simulink model "average_example"  (R2018b)
settings: Solver=ode45  StartTime=0.0  StopTime=24*3600  MaxStep=60  RelTol=1e-3  EnableMultiTasking=on
libraries: carnot x1
settings Model: Creator=drhf  LastModifiedBy=drhf
settings DataIOCC: LimitDataPoints=on  SaveFormat=Array  SignalLoggingSaveFormat=ModelDataLogs
settings OptimizationCC: ExpressionDepthLimit=2147483647  LifeSpan=inf
settings DebuggingCC: UnderspecifiedInitializationDetection=Classic  MergeDetectMultiDrivingBlocksExec=none  SolverPrmCheckMsg=warning  FcnCallInpInsideContextMsg=warning  StateNameClashWarn=warning  SFUnexpectedBacktrackingDiag=warning  SFNoUnconditionalDefaultTransitionDiag=warning  SFExecutionAtInitializationDiag=none
settings HardwareCC: ProdBitPerPointer=32  ProdBitPerSizeT=32  ProdBitPerPtrDiffT=32  ProdLargestAtomicFloat=None  ProdIntDivRoundTo=Undefined  ProdEndianess=Unspecified  ProdWordSize=32  ProdHWDeviceType=32-bit Generic
settings ModelReferenceCC: PropagateSignalLabelsOutOfModel=off
settings SFSimCC: SimUseLocalCustomCode=off
settings RTWCC: RTWUseLocalCustomCode=off
settings CodeAppCC: StateflowObjectComments=on
settings GRTTargetCC: TargetLangStandard=C89/C90 (ANSI)  GeneratePreprocessorConditionals=Disable all  CombineOutputUpdateFcns=off  GRTInterface=on
settings ConfigComp: CovMetricSettings=dw  CovHtmlReporting=on  CovSaveCumulativeToWorkspaceVar=on  CovSaveSingleToWorkspaceVar=on  CovExternalEMLEnable=off

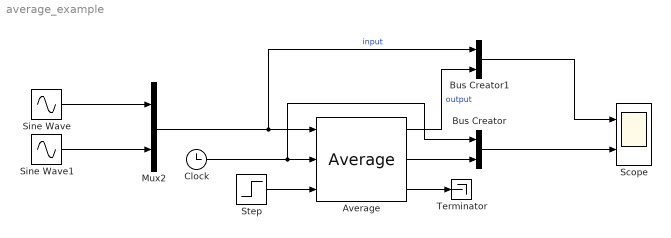
== system average_example ==
  Average : carnot/Toolbox/Average  time_intervall=3600  offset_flag=on  enable_flag=on
      settings: SourceProductName=Carnot
  Bus Creator : BusCreator  Inputs=2
  Bus Creator1 : BusCreator  Inputs=2
  Clock : Clock
  Mux2 : Mux  Inputs=2
  Scope : Scope  NumInputPorts=2
  Sine Wave : Sin  Frequency=2*pi/(24*3600)  SampleTime=0
  Sine Wave1 : Sin  Frequency=2*pi/(24*3600)  Phase=3*3600  SampleTime=0
  Step : Step  Time=2*3600  SampleTime=0
  Terminator : Terminator
  wires:
  Sine Wave/1 -> Mux2/1
  Clock/1 -> Bus Creator/1, Average/2
  Step/1 -> Average/3
  Average/2 -> Bus Creator/2
  Average/1 -> Bus Creator1/2  "output"
  Mux2/1 -> Bus Creator1/1, Average/1  "input"
  Sine Wave1/1 -> Mux2/2
  Bus Creator1/1 -> Scope/1
  Average/3 -> Terminator/1
  Bus Creator/1 -> Scope/2
